simulink subsystem "Global_Line_Divide"  (R2022b)
settings: Solver=VariableStepAuto  StartTime=0.0  StopTime=10.0  RelTol=1e-3
settings Model: Creator=User  LastModifiedBy=User

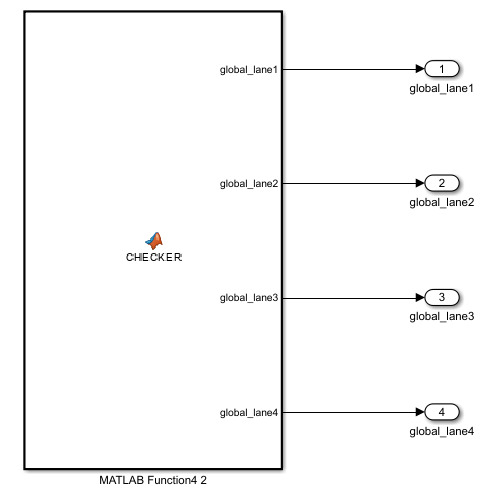
[thumbnail: Simulink's stored preview of the top-level diagram]
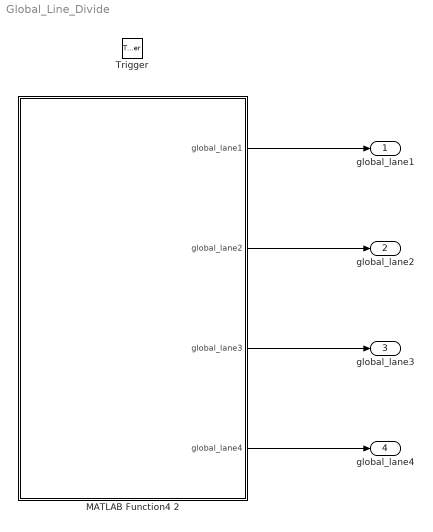
== system Global_Line_Divide ==
  Trigger : TriggerPort  VariantControl=(inherit)  PortDimensions=1
  MATLAB Function4 2 : MATLAB Function  TreatAsAtomicUnit=on
  global_lane1 : Outport
  global_lane2 : Outport  Port=2
  global_lane3 : Outport  Port=3
  global_lane4 : Outport  Port=4
  wires:
  MATLAB Function4 2/1(global_lane1) -> global_lane1/1
  MATLAB Function4 2/2(global_lane2) -> global_lane2/1
  MATLAB Function4 2/3(global_lane3) -> global_lane3/1
  MATLAB Function4 2/4(global_lane4) -> global_lane4/1

== matlab function Global_Line_Divide/MATLAB Function4 2 ==
  settings: sampleTime=0.1
  data: global_lane1 output; global_lane2 output; global_lane3 output; global_lane4 output
function [global_lane1, global_lane2, global_lane3, global_lane4] = CHECKER()

    %% Localization plotter
    f1 = load('waypoints_data.mat');
    f2 = load('roadprofiles_data.mat');

    n_waypoint = height(f1.ids);
    n_roadprofile = height(f2.ids);

    % 미리 고정된 크기의 큰 배열로 초기화
    max_size = 1000; % 필요에 따라 적절한 값으로 설정
    global_lane1 = NaN(max_size, 2); % NaN으로 초기화하여 미리 고정 크기를 설정
    global_lane2 = NaN(max_size, 2);
    global_lane3 = NaN(max_size, 2);
    global_lane4 = NaN(max_size, 2);

    lane1_idx = 1;
    lane2_idx = 1;
    lane3_idx = 1;
    lane4_idx = 1;

    % Loop through each road profile
    for i = 1 : n_roadprofile
        x = zeros(1, 50);
        y = zeros(1, 50);
        idx = 1;

        for j = 1:50
            if f2.waypoints(i,j) ~= 0
                x(idx) = f1.waypoints(f2.waypoints(i,j),1);
                y(idx) = f1.waypoints(f2.waypoints(i,j),2);

                if x(idx) >= -200 && x(idx) <= 200 && y(idx) >= -200 && y(idx) <= 200
                    idx = idx + 1;
                end
            end
        end

        % 유효한 값을 각 lane에 추가
        if ismember(i, 1:10)
            global_lane1(lane1_idx:lane1_idx+idx-2, :) = [x(1:idx-1)', y(1:idx-1)'];
            lane1_idx = lane1_idx + idx - 1;
        elseif ismember(i, 11:20)
            global_lane2(lane2_idx:lane2_idx+idx-2, :) = [x(1:idx-1)', y(1:idx-1)'];
            lane2_idx = lane2_idx + idx - 1;
        elseif ismember(i, 21:30)
            global_lane3(lane3_idx:lane3_idx+idx-2, :) = [x(1:idx-1)', y(1:idx-1)'];
            lane3_idx = lane3_idx + idx - 1;
        elseif ismember(i, 31:33)
            global_lane4(lane4_idx:lane4_idx+idx-2, :) = [x(1:idx-1)', y(1:idx-1)'];
            lane4_idx = lane4_idx + idx - 1;
        end
    end

    % 더 이상 할당할 필요 없이 global_lane을 그대로 사용
end
